simulink model "MPC"  (R2016a)
settings: Solver=VariableStepAuto  StartTime=0.0  StopTime=10  RelTol=1e-3
values from neighbouring files (symbols this model uses):
  ba = 3e-4    (= 0.0003)    [Ini_non_lin.m]
  bl = 0.001    [Ini_non_lin.m]
  Jm = 6.375e-04    (= 0.0006375)    [Ini_non_lin.m]
  kb = 4.875    [Ini_non_lin.m]
  Ke = 0.0169    [Ini_non_lin.m]
  ks = 48.75    [Ini_non_lin.m]
  Kt = 191.3    [Ini_non_lin.m]
  l = 80e-3    (= 0.08)    [Ini_non_lin.m]
  Ld = 3.427e-3    (= 0.003427)    [Ini_non_lin.m]
  Lq = 3.334e-3    (= 0.003334)    [Ini_non_lin.m]
  M = 10    [Ini_non_lin.m]
  p = 6    [Ini_non_lin.m]    (also in The_whole_system_conected.m = 50)
  q = 9e-3    (= 0.009)    [Ini_non_lin.m]
  r = 22.5e-3    (= 0.0225)    [Ini_non_lin.m]
  R = 378e-3    (= 0.378)    [Ini_non_lin.m]
libraries: mpclib x1
settings Model: Creator=Loki  LastModifiedBy=Loki
settings DataIOCC: LimitDataPoints=on
settings DebuggingCC: AllowSymbolicDim=off
settings ModelReferenceCC: PropagateSignalLabelsOutOfModel=off
settings GRTTargetCC: GeneratePreprocessorConditionals=Use local settings

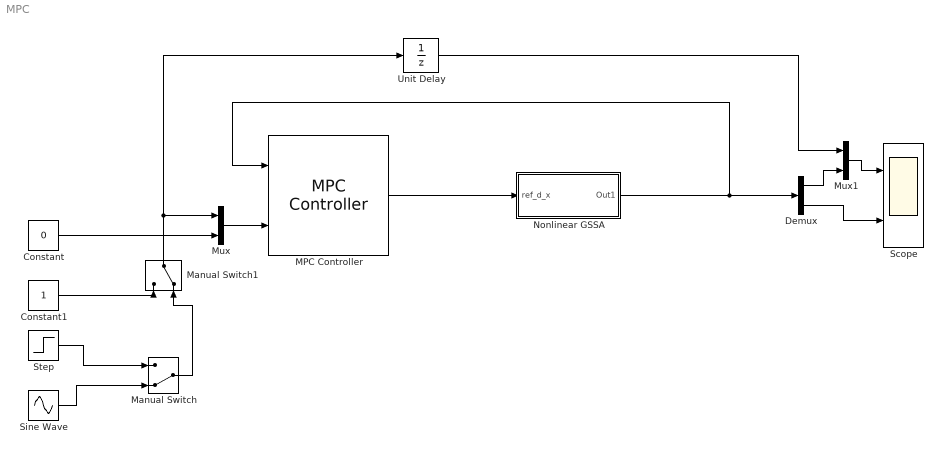
== system MPC ==
  Constant : Constant  Value=0  SampleTime=0.001
  Constant1 : Constant  SampleTime=0.001
  Demux : Demux  Outputs=2
  MPC Controller : mpclib/MPC Controller  SCDEnableBlockLinearizationSpecification=on  mpcobj=MPCobj  is_multiple=0  enable_value=0  return_u0=off  ref_from_ws=off  ref_signal_name=[]  ref_preview=off  md_from_ws=off  md_signal_name=[]  md_preview=off  from_project=off  project_file=MPCtask.mat  md_inport=off  mv_inport=off  cost_outport=off  return_sequence=off  return_qpstatus=off  return_state=off  state_inport=off  lims_inport=off  ywt_inport=off  is_designfromscratch=0  uwt_inport=off  duwt_inport=off  rhoeps_inport=off  uref_inport=off  n_ts=0.001  n_mv=1  n_md=0  n_ud=0  n_mo=2  n_uo=1  BlockDataType=double  SampleTimeInherited=off  switch_inport=off
  Manual Switch : ManualSwitch  CurrentSetting=0
  Manual Switch1 : ManualSwitch  CurrentSetting=0
  Mux : Mux  Inputs=2
  Mux1 : Mux  Inputs=2
  Nonlinear GSSA : Subsystem
  Scope : Scope  NumInputPorts=2
  Sine Wave : Sin  Amplitude=8  Frequency=6.28
  Step : Step
  Unit Delay : UnitDelay  SampleTime=-1
  wires:
  Step/1 -> Manual Switch/1
  Sine Wave/1 -> Manual Switch/2
  Demux/2 -> Scope/2
  Mux/1 -> MPC Controller/2
  Constant/1 -> Mux/2
  Mux1/1 -> Scope/1
  Demux/1 -> Mux1/2
  Unit Delay/1 -> Mux1/1
  Manual Switch/1 -> Manual Switch1/2
  Manual Switch1/1 -> Unit Delay/1, Mux/1
  Constant1/1 -> Manual Switch1/1
  MPC Controller/1 -> Nonlinear GSSA/1(ref_d_x)
  Nonlinear GSSA/1(Out1) -> MPC Controller/1, Demux/1

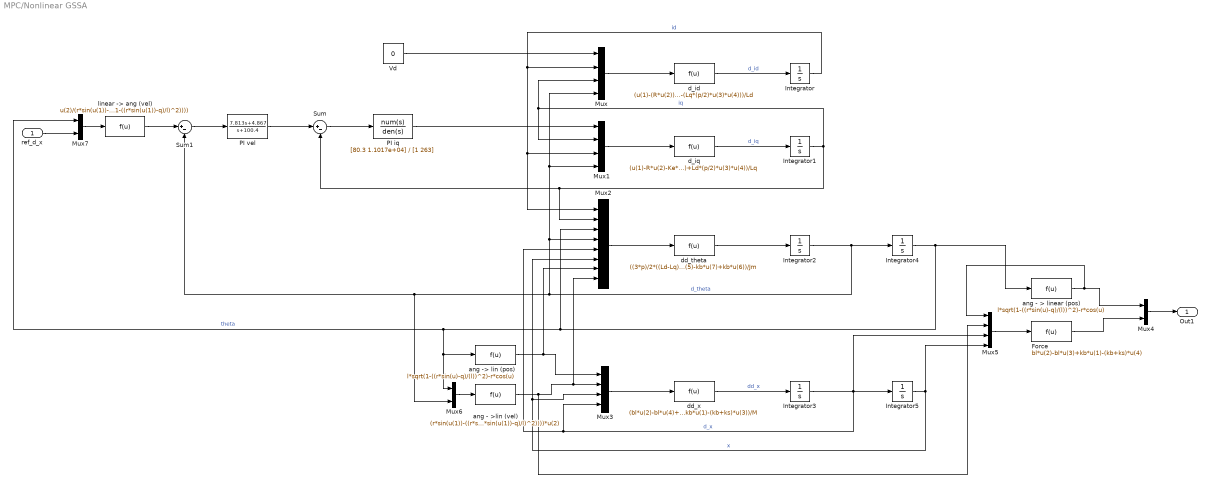
== system MPC/Nonlinear GSSA ==
  ref_d_x : Inport
  Force : Fcn  Expr=bl*u(2)-bl*u(3)+kb*u(1)-(kb+ks)*u(4)
  Integrator{,1..5} (6 alike) : Integrator
  Mux{,1,3,5} (4 alike) : Mux
  Mux2 : Mux  Inputs=8
  Mux4 : Mux  Inputs=2
  Mux6 : Mux  Inputs=2
  Mux7 : Mux  Inputs=2
  PI iq : TransferFcn  Numerator=[80.3 1.1017e+04]  Denominator=[1 263]
  PI vel : TransferFcn  Numerator=[7.813 4.867]  Denominator=[1 100.4]
  Sum : Sum  Inputs=|+-
  Sum1 : Sum  Inputs=|+-
  Vd : Constant  Value=0
  ang - > linear (pos) : Fcn  Expr=l*sqrt(1-((r*sin(u)-q)/(l))^2)-r*cos(u)
  ang - >lin (vel) : Fcn  Expr=(r*sin(u(1))-((r*sin(u(1))*cos(u(1))-r*q*cos(u(1)))/(l*sqrt(1-((r*sin(u(1))-q)/l)^2))))*u(2)
  "ang -> lin (pos)" : Fcn  Expr=l*sqrt(1-((r*sin(u)-q)/(l))^2)-r*cos(u)
  d_id : Fcn  Expr=(u(1)-(R*u(2))-(Lq*(p/2)*u(3)*u(4)))/Ld
  d_iq : Fcn  Expr=(u(1)-R*u(2)-Ke*u(4)+Ld*(p/2)*u(3)*u(4))/Lq
  dd_theta : Fcn  Expr=((3*p)/2*((Ld-Lq)*u(1)*u(2))+Kt*u(2)-ba*u(4)-(ba+bl)*u(8)+bl*u(5)-kb*u(7)+kb*u(6))/Jm
  dd_x : Fcn  Expr=(bl*u(2)-bl*u(4)+kb*u(1)-(kb+ks)*u(3))/M
  "linear -> ang (vel)" : Fcn  Expr=u(2)/(r*sin(u(1))-((r*sin(u(1))*cos(u(1))-r*q*cos(u(1)))/(l*sqrt(1-((r*sin(u(1))-q)/l)^2))))
  Out1 : Outport
  wires:
  Integrator2/1 -> Mux1/4, Mux/4, Mux2/4, Mux6/2, Sum1/2, Integrator4/1  "d_theta"
  Mux4/1 -> Out1/1
  PI iq/1 -> Mux1/1
  Vd/1 -> Mux/1
  d_id/1 -> Integrator/1  "d_id"
  Mux1/1 -> d_iq/1
  d_iq/1 -> Integrator1/1  "d_iq"
  dd_theta/1 -> Integrator2/1
  Mux2/1 -> dd_theta/1
  Mux3/1 -> dd_x/1
  dd_x/1 -> Integrator3/1  "dd_x"
  Mux/1 -> d_id/1
  Sum/1 -> PI iq/1
  PI vel/1 -> Sum/1
  "linear -> ang (vel)"/1 -> Sum1/1
  Sum1/1 -> PI vel/1
  Integrator1/1 -> Mux2/2, Sum/2, Mux/3, Mux1/2  "iq"
  ang - > linear (pos)/1 -> Mux5/1, Mux4/1
  Force/1 -> Mux4/2
  Integrator/1 -> Mux/2, Mux2/1, Mux1/3  "id"
  Integrator5/1 -> Mux3/3, Mux2/6, Mux5/4  "x"
  Integrator3/1 -> Mux3/4, Mux2/5, Integrator5/1, Mux5/3  "d_x"
  Integrator4/1 -> Mux7/1, "ang -> lin (pos)"/1, Mux6/1, Mux2/3, ang - > linear (pos)/1  "theta"
  Mux5/1 -> Force/1
  ang - >lin (vel)/1 -> Mux5/2, Mux2/8, Mux3/2
  Mux6/1 -> ang - >lin (vel)/1
  "ang -> lin (pos)"/1 -> Mux2/7, Mux3/1
  Mux7/1 -> "linear -> ang (vel)"/1
  ref_d_x/1 -> Mux7/2
